simulink model "MMSimulink"  (R2022b)
settings: Solver=VariableStepAuto  StartTime=0.0  StopTime=2000  RelTol=1e-3
values from neighbouring files (symbols this model uses):
  EK = (R*T)/F*log(Ko / Ki)    [RunMe.m]
  G = 0.0376    [RunMe.m]
  Vm = Vm_values(i)    [RunMe.m]
settings Model: Creator=Utente  LastModifiedBy=Utente

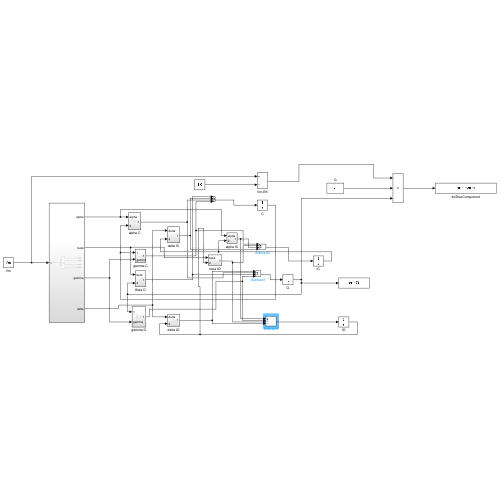
[thumbnail: Simulink's stored preview of the top-level diagram]
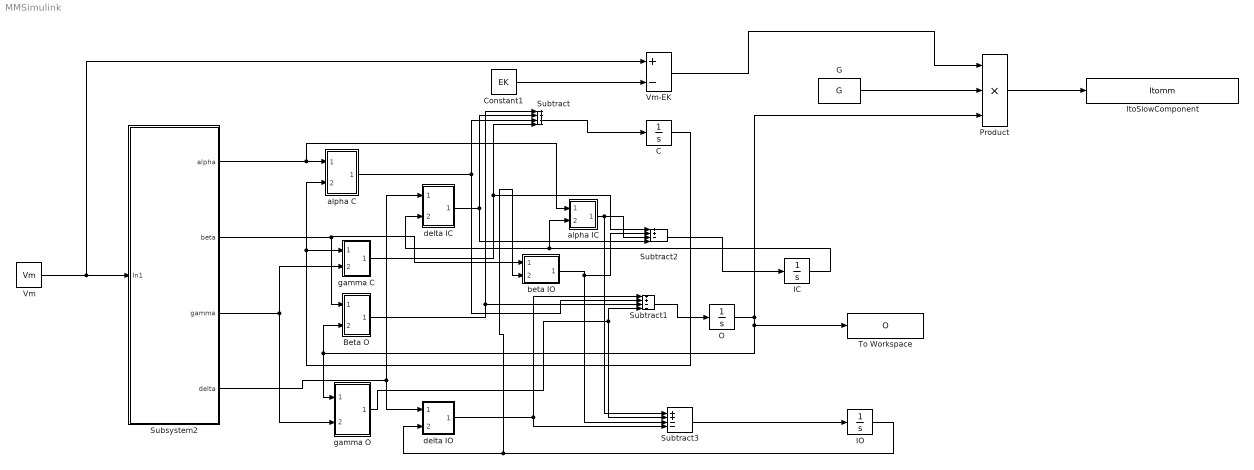
== system MMSimulink ==
  Beta O : Subsystem
  C : Integrator  InitialCondition=1
  Constant1 : Constant  Value=EK
  G : Constant  Value=G
  IC : Integrator
  IO : Integrator
  ItoSlowComponent : ToWorkspace  VariableName=Itomm  SampleTime=-1
  O : Integrator
  Product : Product  Inputs=3
  Subsystem2 : Subsystem
  Subtract{,1..3} (4 alike) : Sum  Inputs=++--
  To Workspace : ToWorkspace  VariableName=O  SampleTime=-1
  Vm : Constant  Value=Vm
  Vm-EK : Sum  Inputs=+-
  alpha C : Subsystem
  alpha IC : Subsystem
  beta IO : Subsystem
  delta IC : Subsystem
  delta IO : Subsystem
  gamma C : Subsystem
  gamma O : Subsystem
  wires:
  Subsystem2/4(delta) -> delta IC/1(delta), delta IO/1(delta)
  Vm/1 -> Vm-EK/1, Subsystem2/1(In1)
  Constant1/1 -> Vm-EK/2
  Vm-EK/1 -> Product/1
  G/1 -> Product/2
  Product/1 -> ItoSlowComponent/1
  Subsystem2/1(alpha) -> alpha IC/1(alpha), alpha C/1(alpha)
  C/1 -> alpha C/2(In2), gamma C/1(In1)
  Subsystem2/3(gamma) -> gamma C/2(gamma), gamma O/2(gamma)
  IC/1 -> alpha IC/2(In2), delta IC/2(In2)
  Subsystem2/2(beta) -> beta IO/1(beta), Beta O/1(beta)
  O/1 -> Product/3, To Workspace/1, gamma O/1(In1), Beta O/2(In2)
  Beta O/1(Out1) -> Subtract/1, Subtract1/3
  delta IC/1(Out1) -> Subtract/2, Subtract2/4
  alpha C/1(Out1) -> Subtract1/2, Subtract/3
  gamma C/1(Out1) -> Subtract/4, Subtract2/1
  Subtract/1 -> C/1
  IO/1 -> beta IO/2(In2), delta IO/2(In2)
  delta IO/1(Out1) -> Subtract3/4, Subtract1/1
  gamma O/1(Out1) -> Subtract3/2, Subtract1/4
  beta IO/1(Out1) -> Subtract3/3, Subtract2/2
  alpha IC/1(Out1) -> Subtract3/1, Subtract2/3
  Subtract2/1 -> IC/1
  Subtract1/1 -> O/1
  Subtract3/1 -> IO/1

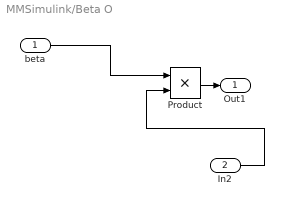
== system MMSimulink/Beta O ==
  beta : Inport
  In2 : Inport  Port=2
  Product : Product
  Out1 : Outport
  wires:
  beta/1 -> Product/1
  Product/1 -> Out1/1
  In2/1 -> Product/2

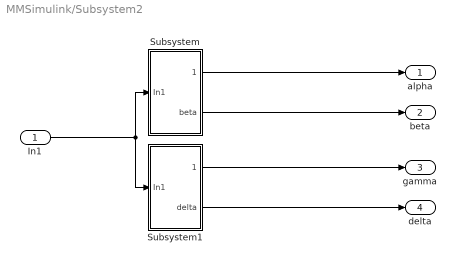
== system MMSimulink/Subsystem2 ==
  In1 : Inport
  Subsystem : Subsystem
  Subsystem1 : Subsystem
  alpha : Outport
  beta : Outport  Port=2
  gamma : Outport  Port=3
  delta : Outport  Port=4
  wires:
  Subsystem1/1(gamma) -> gamma/1
  In1/1 -> Subsystem/1(In1), Subsystem1/1(In1)
  Subsystem/1(alpha) -> alpha/1
  Subsystem1/2(delta) -> delta/1
  Subsystem/2(beta) -> beta/1

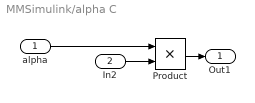
== system MMSimulink/alpha C ==
  alpha : Inport
  In2 : Inport  Port=2
  Product : Product
  Out1 : Outport
  wires:
  Product/1 -> Out1/1
  alpha/1 -> Product/1
  In2/1 -> Product/2

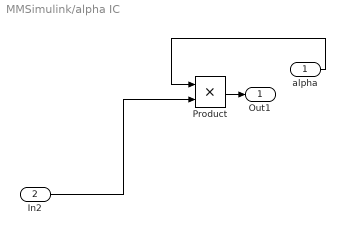
== system MMSimulink/alpha IC ==
  alpha : Inport
  In2 : Inport  Port=2
  Product : Product
  Out1 : Outport
  wires:
  alpha/1 -> Product/1
  Product/1 -> Out1/1
  In2/1 -> Product/2

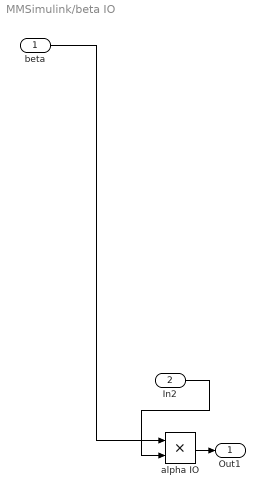
== system MMSimulink/beta IO ==
  beta : Inport
  In2 : Inport  Port=2
  alpha IO : Product
  Out1 : Outport
  wires:
  In2/1 -> alpha IO/2
  alpha IO/1 -> Out1/1
  beta/1 -> alpha IO/1

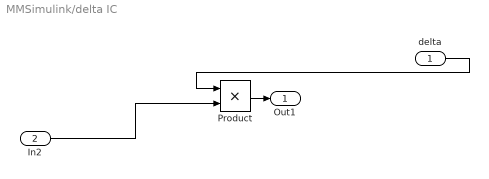
== system MMSimulink/delta IC ==
  delta : Inport
  In2 : Inport  Port=2
  Product : Product
  Out1 : Outport
  wires:
  delta/1 -> Product/1
  In2/1 -> Product/2
  Product/1 -> Out1/1

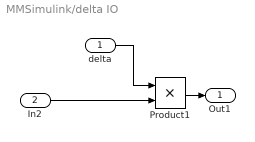
== system MMSimulink/delta IO ==
  delta : Inport
  In2 : Inport  Port=2
  Product1 : Product
  Out1 : Outport
  wires:
  delta/1 -> Product1/1
  Product1/1 -> Out1/1
  In2/1 -> Product1/2

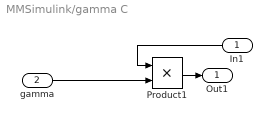
== system MMSimulink/gamma C ==
  In1 : Inport
  gamma : Inport  Port=2
  Product1 : Product
  Out1 : Outport
  wires:
  In1/1 -> Product1/1
  gamma/1 -> Product1/2
  Product1/1 -> Out1/1

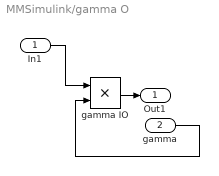
== system MMSimulink/gamma O ==
  In1 : Inport
  gamma : Inport  Port=2
  gamma IO : Product
  Out1 : Outport
  wires:
  gamma IO/1 -> Out1/1
  gamma/1 -> gamma IO/2
  In1/1 -> gamma IO/1

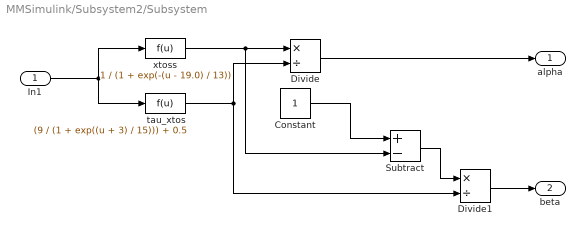
== system MMSimulink/Subsystem2/Subsystem ==
  In1 : Inport
  Constant : Constant
  Divide : Product  Inputs=*/  RndMeth=Zero  SaturateOnIntegerOverflow=on
  Divide1 : Product  Inputs=*/  RndMeth=Zero  SaturateOnIntegerOverflow=on
  Subtract : Sum  Inputs=+-
  tau_xtos : Fcn  Expr=(9 / (1 + exp((u + 3) / 15))) + 0.5
  xtoss : Fcn  Expr=1 / (1 + exp(-(u - 19.0) / 13))
  alpha : Outport
  beta : Outport  Port=2
  wires:
  In1/1 -> tau_xtos/1, xtoss/1
  Subtract/1 -> Divide1/1
  tau_xtos/1 -> Divide1/2, Divide/2
  xtoss/1 -> Subtract/2, Divide/1
  Divide/1 -> alpha/1
  Constant/1 -> Subtract/1
  Divide1/1 -> beta/1

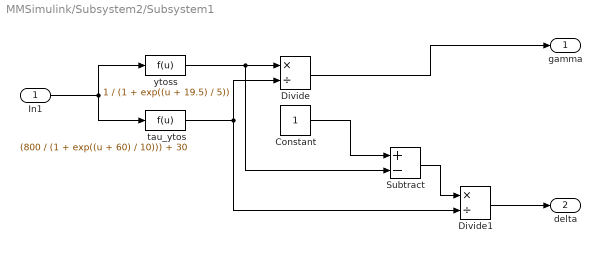
== system MMSimulink/Subsystem2/Subsystem1 ==
  In1 : Inport
  Constant : Constant
  Divide : Product  Inputs=*/  RndMeth=Zero  SaturateOnIntegerOverflow=on
  Divide1 : Product  Inputs=*/  RndMeth=Zero  SaturateOnIntegerOverflow=on
  Subtract : Sum  Inputs=+-
  tau_ytos : Fcn  Expr=(800 / (1 + exp((u + 60) / 10))) + 30
  ytoss : Fcn  Expr=1 / (1 + exp((u + 19.5) / 5))
  gamma : Outport
  delta : Outport  Port=2
  wires:
  In1/1 -> tau_ytos/1, ytoss/1
  ytoss/1 -> Subtract/2, Divide/1
  tau_ytos/1 -> Divide1/2, Divide/2
  Constant/1 -> Subtract/1
  Divide/1 -> gamma/1
  Subtract/1 -> Divide1/1
  Divide1/1 -> delta/1
